simulink model "sim_taes_2023_att"  (R2020a)
settings: Solver=ode4  StartTime=0.0  StopTime=30.0  FixedStep=0.01  RelTol=1e-3
values from neighbouring files (symbols this model uses):
  c1_diff_sigma_bar_w = diag([12; 12; 12])    [init_taes_2023_att.m]
  c1_diff_ui = diag([25; 30; 20])    [init_taes_2023_att.m]
  c2_diff_sigma_bar_w = diag([12; 12; 12])    [init_taes_2023_att.m]
  c2_diff_ui = diag([50; 50; 10])    [init_taes_2023_att.m]
  c3_diff_sigma_bar_w = diag([15; 15; 15])    [init_taes_2023_att.m]
  c3_diff_ui = diag([15; 15; 10])    [init_taes_2023_att.m]
  cw = diag([4.0; 4.0; 4.0])    [init_taes_2023_att.m]
  dw_aa_t = 0.2 * ones(3, 5) + ( 1.0 - 0.2 ) * rand(3, 5)    [init_taes_2023_att.m]
  dw_ff_t = [ 0.4 * ones(1, 5) + ( 1.0 - 0.4 ) * rand(1, 5);                      0.4 * ones(1, 5) + ( 1.0 - 0.4 ) * rand(1, 5);                      0.2 * ones(1, 5) + ( 0.6 - 0.2 ) * rand(1, 5) ]    [init_taes_2023_att.m]
  dw_phi_t = ( - pi / 2 ) * ones(3, 5) + ( pi / 2 - ( - pi / 2 ) ) * rand(3, 5)    [init_taes_2023_att.m]
  dwci_init = zeros(3,5)    [init_taes_2023_att.m]
  h1w = diag([20.0; 20.0; 20.0])    [init_taes_2023_att.m]
  h2w = diag([35.0; 35.0; 35.0])    [init_taes_2023_att.m]
  h3w = diag([30.0; 30.0; 30.0])    [init_taes_2023_att.m]
  Ji = zeros(3,3,NF)    [init_taes_2023_att.m]
  kR = diag([40; 40; 40])    [init_taes_2023_att.m]
  kRtilt = diag([90; 90; 90])    [init_taes_2023_att.m]
  Lamd_diff_sigma_bar_w = 0.5    [init_taes_2023_att.m]
  Lamd_diff_ui = 0.5    [init_taes_2023_att.m]
  mu_d_w = 100    [init_taes_2023_att.m]
  pos0 = zeros(3, 1)    [init_taes_2023_att.m]
  PZ0 = P0(3)    [init_taes_2023_att.m]
  PZ1 = 10    [init_taes_2023_att.m]
  Qci_init = repmat([1;0;0;0],1,NF)    [init_taes_2023_att.m]
  R0 = 4    [init_taes_2023_att.m]
  R1 = 8    [init_taes_2023_att.m]
  Rci_init = zeros(3,3,NF)    [init_taes_2023_att.m]
  Ri_init = zeros(3,3,NF)    [init_taes_2023_att.m]
  Rx2 = 10    [init_taes_2023_att.m]
  Ry2 = 6    [init_taes_2023_att.m]
  Rz2 = 4    [init_taes_2023_att.m]
  T0 = 0    [init_taes_2023_att.m]
  T1 = tseq1    (= 10)    [init_taes_2023_att.m]
  T2 = tseq1 + tseq12 + tseq2    (= 30)    [init_taes_2023_att.m]
  ui_init = zeros(3,NF)    [init_taes_2023_att.m]
  vel0 = zeros(3, 1)    [init_taes_2023_att.m]
  wci_init = zeros(3,5)    [init_taes_2023_att.m]
  zeta_diff_sigma_bar_w = 0.08    [init_taes_2023_att.m]
  zeta_diff_ui = 0.08    [init_taes_2023_att.m]
undefined symbols (not defined in the file or in its folder): cal_frac_squ, p_alfaw1, p_alfaw2, q_alfaw1, q_alfaw2, Qei_init, Qeitilt_init, Qi_init, Rei_init, Reitilt_init, V_Phi_Rei_init, V_Phi_Reitilt_init, wei_init, weitilt_init, wi_init
(part 4 of 4)

== matlab function sim_taes_2023_att/cal Ri agent 5 ==
  data: Ri_5 output; Qi_vec input
function Ri_5 = fcn(Qi_vec)
%%%% 使用罗德里格公式由四元数Qi求解Ri
iiuav = 5;
thetai_tmp = Qi_vec(1,iiuav);
qi_tmp = Qi_vec(2:4,iiuav);
Ri_5 = ((thetai_tmp^2) - (qi_tmp')*qi_tmp) * eye(3,3) ...
            + 2 * qi_tmp * (qi_tmp') ...
            - 2 * thetai_tmp * cal_askew_mat(qi_tmp);

end

== matlab function sim_taes_2023_att/cal Qci agent 1 ==
  data: Qi_vec input; Qci_1 output; Qei_vec input
function Qci_1 = fcn(Qi_vec, Qei_vec)
%%%% 更新期望指令四元数
iiuav = 1;

sigma1 = Qi_vec(1,iiuav);
q1 = Qi_vec(2:4,iiuav);
sigma2 = Qei_vec(1,iiuav);
q2 = -Qei_vec(2:4,iiuav);

sigma = sigma1*sigma2 - (q1')*q2;
q = sigma1*q2 + sigma2*q1 + cal_askew_mat(q1)*q2;
Qci_1 = [sigma; q];

end

== matlab function sim_taes_2023_att/cal Rci agent 1 ==
  data: Rci_1 output; Qci input
function Rci_1 = fcn(Qci)
%%%% 使用罗德里格公式由四元数Qci求解Rci
thetaci_tmp = Qci(1,1);
qci_tmp = Qci(2:4,1);
Rci_1 = ((thetaci_tmp^2) - (qci_tmp')*qci_tmp) * eye(3,3) ...
                + 2 * qci_tmp * (qci_tmp') ...
                - 2 * thetaci_tmp * cal_askew_mat(qci_tmp);

end

== matlab function sim_taes_2023_att/cal Qci agent 2 ==
  data: Qi_vec input; Qci_2 output; Qei_vec input
function Qci_2 = fcn(Qi_vec, Qei_vec)
%%%% 更新期望指令四元数
iiuav = 2;
sigma1 = Qi_vec(1,iiuav);
q1 = Qi_vec(2:4,iiuav);
sigma2 = Qei_vec(1,iiuav);
q2 = -Qei_vec(2:4,iiuav);

sigma = sigma1*sigma2 - (q1')*q2;
q = sigma1*q2 + sigma2*q1 + cal_askew_mat(q1)*q2;
Qci_2 = [sigma; q];

end

== matlab function sim_taes_2023_att/cal Rci agent 2 ==
  data: Rci_2 output; Qci input
function Rci_2 = fcn(Qci)
%%%% 使用罗德里格公式由四元数Qci求解Rci

thetaci_tmp = Qci(1,1);
qci_tmp = Qci(2:4,1);
Rci_2 = ((thetaci_tmp^2) - (qci_tmp')*qci_tmp) * eye(3,3) ...
                + 2 * qci_tmp * (qci_tmp') ...
                - 2 * thetaci_tmp * cal_askew_mat(qci_tmp);

end

== matlab function sim_taes_2023_att/cal Qci agent 3 ==
  data: Qi_vec input; Qci_3 output; Qei_vec input
function Qci_3 = fcn(Qi_vec, Qei_vec)
%%%% 更新期望指令四元数
iiuav = 3;
sigma1 = Qi_vec(1,iiuav);
q1 = Qi_vec(2:4,iiuav);
sigma2 = Qei_vec(1,iiuav);
q2 = -Qei_vec(2:4,iiuav);

sigma = sigma1*sigma2 - (q1')*q2;
q = sigma1*q2 + sigma2*q1 + cal_askew_mat(q1)*q2;
Qci_3 = [sigma; q];

end

== matlab function sim_taes_2023_att/cal differentiator d_sigma_bar_w_hat agent 1/cal sig3 ==
  data: x input; z output; y input
function z = fcn(x, y)
z = x(:) .* sign(y(:));

== matlab function sim_taes_2023_att/cal Rci agent 3 ==
  data: Rci_3 output; Qci input
function Rci_3 = fcn(Qci)
%%%% 使用罗德里格公式由四元数Qci求解Rci
thetaci_tmp = Qci(1,1);
qci_tmp = Qci(2:4,1);
Rci_3 = ((thetaci_tmp^2) - (qci_tmp')*qci_tmp) * eye(3,3) ...
                + 2 * qci_tmp * (qci_tmp') ...
                - 2 * thetaci_tmp * cal_askew_mat(qci_tmp);

end

== matlab function sim_taes_2023_att/cal Qci agent 4 ==
  data: Qi_vec input; Qci_4 output; Qei_vec input
function Qci_4 = fcn(Qi_vec, Qei_vec)
%%%% 更新期望指令四元数
iiuav = 4;
sigma1 = Qi_vec(1,iiuav);
q1 = Qi_vec(2:4,iiuav);
sigma2 = Qei_vec(1,iiuav);
q2 = -Qei_vec(2:4,iiuav);

sigma = sigma1*sigma2 - (q1')*q2;
q = sigma1*q2 + sigma2*q1 + cal_askew_mat(q1)*q2;
Qci_4 = [sigma; q];

end

== matlab function sim_taes_2023_att/cal Rci agent 4 ==
  data: Rci_4 output; Qci input
function Rci_4 = fcn(Qci)
%%%% 使用罗德里格公式由四元数Qci求解Rci
thetaci_tmp = Qci(1,1);
qci_tmp = Qci(2:4,1);
Rci_4 = ((thetaci_tmp^2) - (qci_tmp')*qci_tmp) * eye(3,3) ...
                + 2 * qci_tmp * (qci_tmp') ...
                - 2 * thetaci_tmp * cal_askew_mat(qci_tmp);

end

== matlab function sim_taes_2023_att/cal Qci agent 5 ==
  data: Qi_vec input; Qci_5 output; Qei_vec input
function Qci_5 = fcn(Qi_vec, Qei_vec)
%%%% 更新期望指令四元数
iiuav = 5;
sigma1 = Qi_vec(1,iiuav);
q1 = Qi_vec(2:4,iiuav);
sigma2 = Qei_vec(1,iiuav);
q2 = -Qei_vec(2:4,iiuav);

sigma = sigma1*sigma2 - (q1')*q2;
q = sigma1*q2 + sigma2*q1 + cal_askew_mat(q1)*q2;
Qci_5 = [sigma; q];

end

== matlab function sim_taes_2023_att/cal Rci agent 5 ==
  data: Rci_5 output; Qci_vec input
function Rci_5 = fcn(Qci_vec)
%%%% 使用罗德里格公式由四元数Qci求解Rci
thetaci_tmp = Qci_vec(1,1);
qci_tmp = Qci_vec(2:4,1);
Rci_5 = ((thetaci_tmp^2) - (qci_tmp')*qci_tmp) * eye(3,3) ...
                + 2 * qci_tmp * (qci_tmp') ...
                - 2 * thetaci_tmp * cal_askew_mat(qci_tmp);

end

== matlab function sim_taes_2023_att/combine Qci Rci ==
  data: Qci_1 input; Qci_vec output; Qci_2 input; Qci_3 input; Qci_4 input; Qci_5 input; Rci_1 input; Rci_2 input; Rci_3 input; Rci_4 input; Rci_5 input; Rci_vec output
function [Qci_vec, Rci_vec] = fcn(Qci_1, Qci_2, Qci_3, Qci_4, Qci_5, ...
                                                            Rci_1, Rci_2, Rci_3, Rci_4, Rci_5)
%%%% 合并四元数和姿态旋转矩阵
Qci_vec = zeros(4,5);
Qci_vec(:,1) = Qci_1(:);
Qci_vec(:,2) = Qci_2(:);
Qci_vec(:,3) = Qci_3(:);
Qci_vec(:,4) = Qci_4(:);
Qci_vec(:,5) = Qci_5(:);

Rci_vec = zeros(3,3,5);
Rci_vec(:,:,1) = Rci_1;
Rci_vec(:,:,2) = Rci_2;
Rci_vec(:,:,3) = Rci_3;
Rci_vec(:,:,4) = Rci_4;
Rci_vec(:,:,5) = Rci_5;

== matlab function sim_taes_2023_att/Qeitilt dynam agent 1 ==
  data: Qeitilt_vec input; dQeitilt_1 output; weitilt_vec input
function dQeitilt_1 = fcn(Qeitilt_vec, weitilt_vec)
%%%% 更新四元数误差微分方程
iiuav = 1;

weitilt = weitilt_vec(:,iiuav);
thetaeitilt = Qeitilt_vec(1,iiuav);
qeitilt = Qeitilt_vec(2:4,iiuav);

GammaQeitilt = zeros(4,3);
GammaQeitilt(1,:) = -(qeitilt');
GammaQeitilt(2:4,:) = thetaeitilt*eye(3,3) + cal_askew_mat(qeitilt);
dQeitilt_1 = (1/2)*GammaQeitilt*weitilt;

end

== matlab function sim_taes_2023_att/cal Reitilt agent 1 ==
  data: Reitilt_1 output; Qeitilt_vec input
function Reitilt_1 = fcn(Qeitilt_vec)
%%%% 使用罗德里格公式由四元数Qeitilt求解Reitilt
iiuav = 1;
thetaeitilt_tmp = Qeitilt_vec(1,iiuav);
qeitilt_tmp = Qeitilt_vec(2:4,iiuav);
Reitilt_1 = ((thetaeitilt_tmp^2) - (qeitilt_tmp')*qeitilt_tmp) * eye(3,3) ...
                    + 2 * qeitilt_tmp * (qeitilt_tmp') ...
                    - 2 * thetaeitilt_tmp * cal_askew_mat(qeitilt_tmp);

end

== matlab function sim_taes_2023_att/cal weitilt agent 1 ==
  data: wei_vec input; weitilt_1 output; Reitilt_vec input; wbarei_vec input
function weitilt_1 = fcn(wei_vec, Reitilt_vec, wbarei_vec)
%%%% 更新姿态角速率误差
iiuav = 1;
weitilt_1 = wei_vec(:,iiuav) - (Reitilt_vec(:,:,iiuav)') * wbarei_vec(:,iiuav);

end

== matlab function sim_taes_2023_att/cal differentiator d_sigma_bar_w_hat agent 1/cal sig4 ==
  data: x input; z output; y input
function z = fcn(x, y)
z = x(:) .* sign(y(:));

== matlab function sim_taes_2023_att/Qeitilt dynam agent 2 ==
  data: Qeitilt_vec input; dQeitilt_2 output; weitilt_vec input
function dQeitilt_2 = fcn(Qeitilt_vec, weitilt_vec)
%%%% 更新四元数误差微分方程
iiuav = 2;

weitilt = weitilt_vec(:,iiuav);
thetaeitilt = Qeitilt_vec(1,iiuav);
qeitilt = Qeitilt_vec(2:4,iiuav);

GammaQeitilt = zeros(4,3);
GammaQeitilt(1,:) = -(qeitilt');
GammaQeitilt(2:4,:) = thetaeitilt*eye(3,3) + cal_askew_mat(qeitilt);
dQeitilt_2 = (1/2)*GammaQeitilt*weitilt;

end

== matlab function sim_taes_2023_att/cal Reitilt agent 2 ==
  data: Reitilt_2 output; Qeitilt_vec input
function Reitilt_2 = fcn(Qeitilt_vec)
%%%% 使用罗德里格公式由四元数Qeitilt求解Reitilt
iiuav = 2;
thetaeitilt_tmp = Qeitilt_vec(1,iiuav);
qeitilt_tmp = Qeitilt_vec(2:4,iiuav);
Reitilt_2 = ((thetaeitilt_tmp^2) - (qeitilt_tmp')*qeitilt_tmp) * eye(3,3) ...
                    + 2 * qeitilt_tmp * (qeitilt_tmp') ...
                    - 2 * thetaeitilt_tmp * cal_askew_mat(qeitilt_tmp);

end

== matlab function sim_taes_2023_att/cal weitilt agent 2 ==
  data: wei_vec input; weitilt_2 output; Reitilt_vec input; wbarei_vec input
function weitilt_2 = fcn(wei_vec, Reitilt_vec, wbarei_vec)
%%%% 更新姿态角速率误差
iiuav = 2;
weitilt_2 = wei_vec(:,iiuav) - (Reitilt_vec(:,:,iiuav)') * wbarei_vec(:,iiuav);

end

== matlab function sim_taes_2023_att/Qeitilt dynam agent 3 ==
  data: Qeitilt_vec input; dQeitilt_3 output; weitilt_vec input
function dQeitilt_3 = fcn(Qeitilt_vec, weitilt_vec)
%%%% 更新四元数误差微分方程
iiuav = 3;

weitilt = weitilt_vec(:,iiuav);
thetaeitilt = Qeitilt_vec(1,iiuav);
qeitilt = Qeitilt_vec(2:4,iiuav);

GammaQeitilt = zeros(4,3);
GammaQeitilt(1,:) = -(qeitilt');
GammaQeitilt(2:4,:) = thetaeitilt*eye(3,3) + cal_askew_mat(qeitilt);
dQeitilt_3 = (1/2)*GammaQeitilt*weitilt;

end

== matlab function sim_taes_2023_att/cal Reitilt agent 3 ==
  data: Reitilt_3 output; Qeitilt_vec input
function Reitilt_3 = fcn(Qeitilt_vec)
%%%% 使用罗德里格公式由四元数Qeitilt求解Reitilt
iiuav = 3;
thetaeitilt_tmp = Qeitilt_vec(1,iiuav);
qeitilt_tmp = Qeitilt_vec(2:4,iiuav);
Reitilt_3 = ((thetaeitilt_tmp^2) - (qeitilt_tmp')*qeitilt_tmp) * eye(3,3) ...
                    + 2 * qeitilt_tmp * (qeitilt_tmp') ...
                    - 2 * thetaeitilt_tmp * cal_askew_mat(qeitilt_tmp);

end

== matlab function sim_taes_2023_att/cal weitilt agent 3 ==
  data: wei_vec input; weitilt_3 output; Reitilt_vec input; wbarei_vec input
function weitilt_3 = fcn(wei_vec, Reitilt_vec, wbarei_vec)
%%%% 更新姿态角速率误差
iiuav = 3;
weitilt_3 = wei_vec(:,iiuav) - (Reitilt_vec(:,:,iiuav)') * wbarei_vec(:,iiuav);

end

== matlab function sim_taes_2023_att/Qeitilt dynam agent 4 ==
  data: Qeitilt_vec input; dQeitilt_4 output; weitilt_vec input
function dQeitilt_4 = fcn(Qeitilt_vec, weitilt_vec)
%%%% 更新四元数误差微分方程
iiuav = 4;

weitilt = weitilt_vec(:,iiuav);
thetaeitilt = Qeitilt_vec(1,iiuav);
qeitilt = Qeitilt_vec(2:4,iiuav);

GammaQeitilt = zeros(4,3);
GammaQeitilt(1,:) = -(qeitilt');
GammaQeitilt(2:4,:) = thetaeitilt*eye(3,3) + cal_askew_mat(qeitilt);
dQeitilt_4 = (1/2)*GammaQeitilt*weitilt;

end

== matlab function sim_taes_2023_att/cal Reitilt agent 4 ==
  data: Reitilt_4 output; Qeitilt_vec input
function Reitilt_4 = fcn(Qeitilt_vec)
%%%% 使用罗德里格公式由四元数Qeitilt求解Reitilt
iiuav = 4;
thetaeitilt_tmp = Qeitilt_vec(1,iiuav);
qeitilt_tmp = Qeitilt_vec(2:4,iiuav);
Reitilt_4 = ((thetaeitilt_tmp^2) - (qeitilt_tmp')*qeitilt_tmp) * eye(3,3) ...
                    + 2 * qeitilt_tmp * (qeitilt_tmp') ...
                    - 2 * thetaeitilt_tmp * cal_askew_mat(qeitilt_tmp);

end

== matlab function sim_taes_2023_att/cal weitilt agent 4 ==
  data: wei_vec input; weitilt_4 output; Reitilt_vec input; wbarei_vec input
function weitilt_4 = fcn(wei_vec, Reitilt_vec, wbarei_vec)
%%%% 更新姿态角速率误差
iiuav = 4;
weitilt_4 = wei_vec(:,iiuav) - (Reitilt_vec(:,:,iiuav)') * wbarei_vec(:,iiuav);

end

== matlab function sim_taes_2023_att/Qeitilt dynam agent 5 ==
  data: Qeitilt_vec input; dQeitilt_5 output; weitilt_vec input
function dQeitilt_5 = fcn(Qeitilt_vec, weitilt_vec)
%%%% 更新四元数误差微分方程
iiuav = 5;

weitilt = weitilt_vec(:,iiuav);
thetaeitilt = Qeitilt_vec(1,iiuav);
qeitilt = Qeitilt_vec(2:4,iiuav);

GammaQeitilt = zeros(4,3);
GammaQeitilt(1,:) = -(qeitilt');
GammaQeitilt(2:4,:) = thetaeitilt*eye(3,3) + cal_askew_mat(qeitilt);
dQeitilt_5 = (1/2)*GammaQeitilt*weitilt;

end

== matlab function sim_taes_2023_att/cal differentiator d_sigma_bar_w_hat agent 1/cal sig5 ==
  data: x input; z output; y input
function z = fcn(x, y)
z = x(:) .* sign(y(:));

== matlab function sim_taes_2023_att/cal Reitilt agent 5 ==
  data: Reitilt_5 output; Qeitilt_vec input
function Reitilt_5 = fcn(Qeitilt_vec)
%%%% 使用罗德里格公式由四元数Qeitilt求解Reitilt
iiuav = 5;
thetaeitilt_tmp = Qeitilt_vec(1,iiuav);
qeitilt_tmp = Qeitilt_vec(2:4,iiuav);
Reitilt_5 = ((thetaeitilt_tmp^2) - (qeitilt_tmp')*qeitilt_tmp) * eye(3,3) ...
                    + 2 * qeitilt_tmp * (qeitilt_tmp') ...
                    - 2 * thetaeitilt_tmp * cal_askew_mat(qeitilt_tmp);

end

== matlab function sim_taes_2023_att/cal weitilt agent 5 ==
  data: wei_vec input; weitilt_5 output; Reitilt_vec input; wbarei_vec input
function weitilt_5 = fcn(wei_vec, Reitilt_vec, wbarei_vec)
%%%% 更新姿态角速率误差
iiuav = 5;
weitilt_5 = wei_vec(:,iiuav) - (Reitilt_vec(:,:,iiuav)') * wbarei_vec(:,iiuav);

end

== matlab function sim_taes_2023_att/combine weitilt Qeitilt Reitilt ==
  data: weitilt_1 input; weitilt_vec output; weitilt_2 input; weitilt_3 input; weitilt_4 input; weitilt_5 input; Qeitilt_1 input; Qeitilt_2 input; Qeitilt_3 input; Qeitilt_4 input; Qeitilt_5 input; Reitilt_1 input; Reitilt_2 input; Reitilt_3 input; Reitilt_4 input; Reitilt_5 input; Qeitilt_vec output; Reitilt_vec output
function [weitilt_vec, Qeitilt_vec, Reitilt_vec] = fcn(weitilt_1, weitilt_2, weitilt_3, weitilt_4, weitilt_5, ...
                                                                                            Qeitilt_1, Qeitilt_2, Qeitilt_3, Qeitilt_4, Qeitilt_5, ...
                                                                                            Reitilt_1, Reitilt_2, Reitilt_3, Reitilt_4, Reitilt_5)
%%%% 合并辅助姿态角速率误差/辅助四元数误差/辅助姿态旋转矩阵误差
weitilt_vec = zeros(3,5);
weitilt_vec(:,1) = weitilt_1(:);
weitilt_vec(:,2) = weitilt_2(:);
weitilt_vec(:,3) = weitilt_3(:);
weitilt_vec(:,4) = weitilt_4(:);
weitilt_vec(:,5) = weitilt_5(:);

Qeitilt_vec = zeros(4,5);
Qeitilt_vec(:,1) = Qeitilt_1(:);
Qeitilt_vec(:,2) = Qeitilt_2(:);
Qeitilt_vec(:,3) = Qeitilt_3(:);
Qeitilt_vec(:,4) = Qeitilt_4(:);
Qeitilt_vec(:,5) = Qeitilt_5(:);

Reitilt_vec = zeros(3,3,5);
Reitilt_vec(:,:,1) = Reitilt_1;
Reitilt_vec(:,:,2) = Reitilt_2;
Reitilt_vec(:,:,3) = Reitilt_3;
Reitilt_vec(:,:,4) = Reitilt_4;
Reitilt_vec(:,:,5) = Reitilt_5;

== matlab function sim_taes_2023_att/cal error dw_tilt ==
  data: dw_vec input; dw_hat_vec input; dw_tilt_vec output
function dw_tilt_vec = fcn(dw_vec, dw_hat_vec)
%%%% 计算扰动观测误差dw_tilt
dw_tilt_vec = zeros(3,5);
for iiuav = 1:5
    dw_tilt_vec(:,iiuav) = dw_vec(:,iiuav) - dw_hat_vec(:,iiuav);
end

== matlab function sim_taes_2023_att/combine Qci Rci1 ==
  data: V_Phi_Rei_1 input; V_Phi_Rei_vec output; V_Phi_Rei_2 input; V_Phi_Rei_3 input; V_Phi_Rei_4 input; V_Phi_Rei_5 input; V_Phi_Reitilt_1 input; V_Phi_Reitilt_2 input; V_Phi_Reitilt_3 input; V_Phi_Reitilt_4 input; V_Phi_Reitilt_5 input; V_Phi_Reitilt_vec output
function [V_Phi_Rei_vec, V_Phi_Reitilt_vec] = fcn(V_Phi_Rei_1, V_Phi_Rei_2, V_Phi_Rei_3, V_Phi_Rei_4, V_Phi_Rei_5, ...
                                                                                        V_Phi_Reitilt_1, V_Phi_Reitilt_2, V_Phi_Reitilt_3, V_Phi_Reitilt_4, V_Phi_Reitilt_5)
%%%% 合并LogSO3空间的辅助姿态误差向量
V_Phi_Rei_vec = [V_Phi_Rei_1(:), V_Phi_Rei_2(:), V_Phi_Rei_3(:), V_Phi_Rei_4(:), V_Phi_Rei_5(:)];
V_Phi_Reitilt_vec = [V_Phi_Reitilt_1(:), V_Phi_Reitilt_2(:), V_Phi_Reitilt_3(:), V_Phi_Reitilt_4(:), V_Phi_Reitilt_5(:)];

== matlab function sim_taes_2023_att/depart Qe1 ==
  data: y output; x input
function y = fcn(x)
y = x(:,1);

end

== matlab function sim_taes_2023_att/depart Qe2 ==
  data: y output; x input
function y = fcn(x)
y = x(:,2);

end

== matlab function sim_taes_2023_att/cal differentiator d_sigma_bar_w_hat agent 1/trans to column20 ==
  data: x input; y output
function y = fcn(x)
y = x(:);

== matlab function sim_taes_2023_att/depart Qe3 ==
  data: y output; x input
function y = fcn(x)
y = x(:,3);

end

== matlab function sim_taes_2023_att/depart Qe4 ==
  data: y output; x input
function y = fcn(x)
y = x(:,4);

end

== matlab function sim_taes_2023_att/depart Qe5 ==
  data: y output; x input
function y = fcn(x)
y = x(:,5);

end

== matlab function sim_taes_2023_att/depart Qe5tilt ==
  data: y output; x input
function y = fcn(x)
y = x(:,5);

end

== matlab function sim_taes_2023_att/depart Qe1tilt ==
  data: y output; x input
function y = fcn(x)
y = x(:,1);

end

== matlab function sim_taes_2023_att/depart Qe2tilt ==
  data: y output; x input
function y = fcn(x)
y = x(:,2);

end

== matlab function sim_taes_2023_att/depart Qe3tilt ==
  data: y output; x input
function y = fcn(x)
y = x(:,3);

end

== matlab function sim_taes_2023_att/depart Qe4tilt ==
  data: y output; x input
function y = fcn(x)
y = x(:,4);

end

== matlab function sim_taes_2023_att/depart we1 ==
  data: y output; x input
function y = fcn(x)
y = x(:,1);

end

== matlab function sim_taes_2023_att/depart we2 ==
  data: y output; x input
function y = fcn(x)
y = x(:,2);

end

== matlab function sim_taes_2023_att/cal differentiator d_sigma_bar_w_hat agent 1/trans to column23 ==
  data: x input; y output
function y = fcn(x)
y = x(:);

== matlab function sim_taes_2023_att/depart we3 ==
  data: y output; x input
function y = fcn(x)
y = x(:,3);

end

== matlab function sim_taes_2023_att/depart we4 ==
  data: y output; x input
function y = fcn(x)
y = x(:,4);

end

== matlab function sim_taes_2023_att/depart we5 ==
  data: y output; x input
function y = fcn(x)
y = x(:,5);

end

== matlab function sim_taes_2023_att/depart we5tilt ==
  data: y output; x input
function y = fcn(x)
y = x(:,5);

end

== matlab function sim_taes_2023_att/depart we1tilt ==
  data: y output; x input
function y = fcn(x)
y = x(:,1);

end

== matlab function sim_taes_2023_att/depart we2tilt ==
  data: y output; x input
function y = fcn(x)
y = x(:,2);

end

== matlab function sim_taes_2023_att/depart we3tilt ==
  data: y output; x input
function y = fcn(x)
y = x(:,3);

end

== matlab function sim_taes_2023_att/depart we4tilt ==
  data: y output; x input
function y = fcn(x)
y = x(:,4);

end

== matlab function sim_taes_2023_att/depart V_Phi_Re5 ==
  data: y output; x input
function y = fcn(x)
y = x(:,5);

end

== matlab function sim_taes_2023_att/depart V_Phi_Re1 ==
  data: y output; x input
function y = fcn(x)
y = x(:,1);

end

== matlab function sim_taes_2023_att/cal differentiator d_sigma_bar_w_hat agent 2/cal differentiator ==
  data: c1 input; d_sigma_bar_v_hat output; d_dsigma_bar_v_hat output; d_d2sigma_bar_v_hat output; c2 input; c3 input; chi_t input; sigma_bar_v_sig_1 input; sigma_bar_v_sig_2 input; sigma_bar_v_sig_3 input; sigma_bar_v_sig_4 input; sigma_bar_v_sig_5 input; sigma_bar_v_sig_6 input; d_sigma_bar_v_hat input; d2_sigma_bar_v_hat input
function [d_sigma_bar_v_hat, d_dsigma_bar_v_hat, d_d2sigma_bar_v_hat] = fcn(c1, c2, c3, chi_t, sigma_bar_v_sig_1, sigma_bar_v_sig_2, sigma_bar_v_sig_3, ...
                                                                                                                                                sigma_bar_v_sig_4, sigma_bar_v_sig_5, sigma_bar_v_sig_6, d_sigma_bar_v_hat, d2_sigma_bar_v_hat)
d_d2sigma_bar_v_hat = -chi_t .* c1 * sigma_bar_v_sig_1(:) - (1 - chi_t) .* c1 * sigma_bar_v_sig_2(:);
d_dsigma_bar_v_hat = -chi_t .* c2 * sigma_bar_v_sig_3(:) - (1 - chi_t) .* c2 * sigma_bar_v_sig_4(:) + d2_sigma_bar_v_hat(:);
d_sigma_bar_v_hat = -chi_t .* c3 * sigma_bar_v_sig_5(:) - (1 - chi_t) .* c3 * sigma_bar_v_sig_6(:) + d_sigma_bar_v_hat(:);

== matlab function sim_taes_2023_att/depart V_Phi_Re2 ==
  data: y output; x input
function y = fcn(x)
y = x(:,2);

end

== matlab function sim_taes_2023_att/depart V_Phi_Re3 ==
  data: y output; x input
function y = fcn(x)
y = x(:,3);

end

== matlab function sim_taes_2023_att/depart V_Phi_Re4 ==
  data: y output; x input
function y = fcn(x)
y = x(:,4);

end

== matlab function sim_taes_2023_att/depart V_Phi_Re5tilt ==
  data: y output; x input
function y = fcn(x)
y = x(:,5);

end

== matlab function sim_taes_2023_att/depart V_Phi_Re1tilt ==
  data: y output; x input
function y = fcn(x)
y = x(:,1);

end

== matlab function sim_taes_2023_att/depart V_Phi_Re2tilt ==
  data: y output; x input
function y = fcn(x)
y = x(:,2);

end

== matlab function sim_taes_2023_att/depart V_Phi_Re3tilt ==
  data: y output; x input
function y = fcn(x)
y = x(:,3);

end

== matlab function sim_taes_2023_att/depart V_Phi_Re4tilt ==
  data: y output; x input
function y = fcn(x)
y = x(:,4);

end

== matlab function sim_taes_2023_att/depart dw1 dw_hat_1 ==
  data: y1 output; x1 input; x2 input; y2 output
function [y1, y2] = fcn(x1, x2)
iiuav = 1;
y1 = x1(:,iiuav);
y2 = x2(:,iiuav);

end

== matlab function sim_taes_2023_att/depart dw2 dw_hat_2 ==
  data: y1 output; x1 input; x2 input; y2 output
function [y1, y2] = fcn(x1, x2)
iiuav = 2;
y1 = x1(:,iiuav);
y2 = x2(:,iiuav);

end

== matlab function sim_taes_2023_att/depart dw3 dw_hat_3 ==
  data: y1 output; x1 input; x2 input; y2 output
function [y1, y2] = fcn(x1, x2)
iiuav = 3;
y1 = x1(:,iiuav);
y2 = x2(:,iiuav);

end

== matlab function sim_taes_2023_att/depart dw4 dw_hat_4 ==
  data: y1 output; x1 input; x2 input; y2 output
function [y1, y2] = fcn(x1, x2)
iiuav = 4;
y1 = x1(:,iiuav);
y2 = x2(:,iiuav);

end

== matlab function sim_taes_2023_att/depart dw4 dw_hat_1 ==
  data: y1 output; x1 input; x2 input; y2 output
function [y1, y2] = fcn(x1, x2)
iiuav = 4;
y1 = x1(:,iiuav);
y2 = x2(:,iiuav);

end

== matlab function sim_taes_2023_att/depart Qc1 ==
  data: y output; x input
function y = fcn(x)
y = x(:,1);

end

== matlab function sim_taes_2023_att/depart Qc2 ==
  data: y output; x input
function y = fcn(x)
y = x(:,2);

end

== matlab function sim_taes_2023_att/depart Qc3 ==
  data: y output; x input
function y = fcn(x)
y = x(:,3);

end

== matlab function sim_taes_2023_att/depart Qc4 ==
  data: y output; x input
function y = fcn(x)
y = x(:,4);

end

== matlab function sim_taes_2023_att/depart Qc5 ==
  data: y output; x input
function y = fcn(x)
y = x(:,5);

end

== matlab function sim_taes_2023_att/depart wc1 ==
  data: y output; x input
function y = fcn(x)
y = x(:,1);

end

== matlab function sim_taes_2023_att/depart wc2 ==
  data: y output; x input
function y = fcn(x)
y = x(:,2);

end

== matlab function sim_taes_2023_att/depart wc3 ==
  data: y output; x input
function y = fcn(x)
y = x(:,3);

end

== matlab function sim_taes_2023_att/depart wc4 ==
  data: y output; x input
function y = fcn(x)
y = x(:,4);

end

== matlab function sim_taes_2023_att/depart wc5 ==
  data: y output; x input
function y = fcn(x)
y = x(:,5);

end

== matlab function sim_taes_2023_att/combine tau1 ==
  data: dw_1 input; dw_vec output; dw_2 input; dw_3 input; dw_4 input; dw_5 input
function dw_vec = fcn(dw_1, dw_2, dw_3, dw_4, dw_5)
%%%% 合并辅助姿态角速率
dw_vec = [dw_1(:), dw_2(:), dw_3(:), dw_4(:), dw_5(:)];

== matlab function sim_taes_2023_att/generate angular rate disturbance agent 1 ==
  data: dw_1 output; dw_aa_t input; dw_ff_t input; dw_phi_t input; t input
function dw_1 = fcn(dw_aa_t, dw_ff_t, dw_phi_t, t)
%%%% 姿态动力学方程中的扰动项设置
epsil_t = zeros(3, 1);

for kk = 1:5
    epsil_t = epsil_t + dw_aa_t(:, kk) .* sin( 2 * pi * dw_ff_t(:, kk) * t + dw_phi_t(:, kk) );
end

dw_1 = [ epsil_t(1) + 1.6 * sin( 0.4 * t ) + 2.0 * cos( 0.5 * t ) + 1.4 * sin( 0.7 * t ) ...
                + 4 * exp( -0.1 * t ) * sin( 0.8 * t ) + 3 / ( 1 + exp( -0.2 * ( t - 15 ) ) ); ...
                epsil_t(2) + 1.2 * sin( 0.2 * t ) + 3 * cos( 0.4 * t ) + 0.8 * sin( 0.6 * t ) ...
                + 2 * exp( -0.15 * t ) * cos( 1.2 * t ) + 3 / ( 1 + exp( -0.3 * ( t - 25 ) ) ); ...
                epsil_t(3) + 1.8 * sin( 0.2 * t ) + 1.6 * sin( 0.3 * t ) + 1.6 * cos( 0.4 * t ) ...
                + 4 * exp( -0.05 * t ) * sin( 0.5 * t + pi / 4 ) + 3 / ( 1 + exp( -0.5 * ( t - 20 ) ) ) ];

== matlab function sim_taes_2023_att/generate angular rate disturbance agent 2 ==
  data: dw_2 output; dw_aa_t input; dw_ff_t input; dw_phi_t input; t input
function dw_2 = fcn(dw_aa_t, dw_ff_t, dw_phi_t, t)
%%%% 姿态动力学方程中的扰动项设置
epsil_t = zeros(3, 1);

for kk = 1:5
    epsil_t = epsil_t + dw_aa_t(:, kk) .* sin( 2 * pi * dw_ff_t(:, kk) * t + dw_phi_t(:, kk) );
end

dw_2 = [ epsil_t(1) + 1.6 * sin( 0.2 * t ) + 2.0 * cos( 0.3 * t ) + 1.4 * sin( 0.5 * t ) ...
                + 4 * exp( -0.1 * t ) * sin( 0.5 * t ) + 3 / ( 1 + exp( -0.2 * ( t - 15 ) ) ); ...
                epsil_t(2) + 1.2 * sin( 0.1 * t ) + 3 * cos( 0.2 * t ) + 0.8 * sin( 0.4 * t ) ...
                + 2 * exp( -0.15 * t ) * cos( 0.6 * t ) + 3 / ( 1 + exp( -0.3 * ( t - 25 ) ) ); ...
                epsil_t(3) + 1.8 * sin( 0.1 * t ) + 1.6 * sin( 0.2 * t ) + 1.6 * cos( 0.3 * t ) ...
                + 4 * exp( -0.05 * t ) * sin( 0.4 * t + pi / 4 ) + 3 / ( 1 + exp( -0.5 * ( t - 20 ) ) ) ];

== matlab function sim_taes_2023_att/cal differentiator d_sigma_bar_w_hat agent 2/cal sig ==
  data: x input; z output; y input
function z = fcn(x, y)
z = x(:) .* sign(y(:));

== matlab function sim_taes_2023_att/generate angular rate disturbance agent 3 ==
  data: dw_3 output; dw_aa_t input; dw_ff_t input; dw_phi_t input; t input
function dw_3 = fcn(dw_aa_t, dw_ff_t, dw_phi_t, t)
%%%% 姿态动力学方程中的扰动项设置
epsil_t = zeros(3, 1);

for kk = 1:5
    epsil_t = epsil_t + dw_aa_t(:, kk) .* sin( 2 * pi * dw_ff_t(:, kk) * t + dw_phi_t(:, kk) );
end

dw_3 = [ epsil_t(1) + 1.6 * sin( 0.2 * t ) + 2.0 * cos( 0.3 * t ) + 1.4 * sin( 0.5 * t ) ...
                + 4 * exp( -0.1 * t ) * sin( 0.5 * t ) + 3 / ( 1 + exp( -0.2 * ( t - 15 ) ) ); ...
                epsil_t(2) + 1.2 * sin( 0.1 * t ) + 3 * cos( 0.2 * t ) + 0.8 * sin( 0.4 * t ) ...
                + 2 * exp( -0.15 * t ) * cos( 0.6 * t ) + 3 / ( 1 + exp( -0.3 * ( t - 25 ) ) ); ...
                epsil_t(3) + 1.8 * sin( 0.1 * t ) + 1.6 * sin( 0.2 * t ) + 1.6 * cos( 0.3 * t ) ...
                + 4 * exp( -0.05 * t ) * sin( 0.4 * t + pi / 4 ) + 3 / ( 1 + exp( -0.5 * ( t - 20 ) ) ) ];

== matlab function sim_taes_2023_att/generate angular rate disturbance agent 4 ==
  data: dw_4 output; dw_aa_t input; dw_ff_t input; dw_phi_t input; t input
function dw_4 = fcn(dw_aa_t, dw_ff_t, dw_phi_t, t)
%%%% 姿态动力学方程中的扰动项设置
epsil_t = zeros(3, 1);

for kk = 1:5
    epsil_t = epsil_t + dw_aa_t(:, kk) .* sin( 2 * pi * dw_ff_t(:, kk) * t + dw_phi_t(:, kk) );
end

dw_4 = [ epsil_t(1) + 1.6 * sin( 0.2 * t ) + 2.0 * cos( 0.3 * t ) + 1.4 * sin( 0.5 * t ) ...
                + 4 * exp( -0.1 * t ) * sin( 0.5 * t ) + 3 / ( 1 + exp( -0.2 * ( t - 15 ) ) ); ...
                epsil_t(2) + 1.2 * sin( 0.1 * t ) + 3 * cos( 0.2 * t ) + 0.8 * sin( 0.4 * t ) ...
                + 2 * exp( -0.15 * t ) * cos( 0.6 * t ) + 3 / ( 1 + exp( -0.3 * ( t - 25 ) ) ); ...
                epsil_t(3) + 1.8 * sin( 0.1 * t ) + 1.6 * sin( 0.2 * t ) + 1.6 * cos( 0.3 * t ) ...
                + 4 * exp( -0.05 * t ) * sin( 0.4 * t + pi / 4 ) + 3 / ( 1 + exp( -0.5 * ( t - 20 ) ) ) ];

== matlab function sim_taes_2023_att/generate angular rate disturbance agent 5 ==
  data: dw_5 output; dw_aa_t input; dw_ff_t input; dw_phi_t input; t input
function dw_5 = fcn(dw_aa_t, dw_ff_t, dw_phi_t, t)
%%%% 姿态动力学方程中的扰动项设置
epsil_t = zeros(3, 1);

for kk = 1:5
    epsil_t = epsil_t + dw_aa_t(:, kk) .* sin( 2 * pi * dw_ff_t(:, kk) * t + dw_phi_t(:, kk) );
end

dw_5 = [ epsil_t(1) + 1.6 * sin( 0.2 * t ) + 2.0 * cos( 0.3 * t ) + 1.4 * sin( 0.5 * t ) ...
                + 4 * exp( -0.1 * t ) * sin( 0.5 * t ) + 3 / ( 1 + exp( -0.2 * ( t - 15 ) ) ); ...
                epsil_t(2) + 1.2 * sin( 0.1 * t ) + 3 * cos( 0.2 * t ) + 0.8 * sin( 0.4 * t ) ...
                + 2 * exp( -0.15 * t ) * cos( 0.6 * t ) + 3 / ( 1 + exp( -0.3 * ( t - 25 ) ) ); ...
                epsil_t(3) + 1.8 * sin( 0.1 * t ) + 1.6 * sin( 0.2 * t ) + 1.6 * cos( 0.3 * t ) ...
                + 4 * exp( -0.05 * t ) * sin( 0.4 * t + pi / 4 ) + 3 / ( 1 + exp( -0.5 * ( t - 20 ) ) ) ];

== matlab function sim_taes_2023_att/combine norminal formation control input ==
  data: ui_1 input; ui_vec output; ui_2 input; ui_3 input; ui_4 input; ui_5 input
function ui_vec = fcn(ui_1, ui_2, ui_3, ui_4, ui_5)
%%%% 合并领导者编队跟踪误差结果
ui_vec = [ui_1(:), ui_2(:), ui_3(:), ui_4(:), ui_5(:)];

== matlab function sim_taes_2023_att/control input generator agent 1 ==
  data: u0 input; ui output
function ui  = fcn(u0)
%%%% 给出领导者参考加速度控制输入
g0 = 9.80663;
e3 = [0;0;1];

ui = g0 * e3 + u0(:);

== matlab function sim_taes_2023_att/control input generator agent 2 ==
  data: u0 input; ui output
function ui  = fcn(u0)
%%%% 给出领导者参考加速度控制输入
g0 = 9.80663;
e3 = [0;0;1];

ui = g0 * e3 + u0(:);

== matlab function sim_taes_2023_att/control input generator agent 3 ==
  data: u0 input; ui output
function ui  = fcn(u0)
%%%% 给出领导者参考加速度控制输入
g0 = 9.80663;
e3 = [0;0;1];

ui = g0 * e3 + u0(:);

== matlab function sim_taes_2023_att/control input generator agent 4 ==
  data: u0 input; ui output
function ui  = fcn(u0)
%%%% 给出领导者参考加速度控制输入
g0 = 9.80663;
e3 = [0;0;1];

ui = g0 * e3 + u0(:);

== matlab function sim_taes_2023_att/control input generator agent 5 ==
  data: u0 input; ui output
function ui  = fcn(u0)
%%%% 给出领导者参考加速度控制输入
g0 = 9.80663;
e3 = [0;0;1];

ui = g0 * e3 + u0(:);

== matlab function sim_taes_2023_att/cal differentiator d_sigma_bar_w_hat agent 2/cal sig1 ==
  data: x input; z output; y input
function z = fcn(x, y)
z = x(:) .* sign(y(:));

== matlab function sim_taes_2023_att/cal differentiator d_sigma_bar_w_hat agent 2/cal sig2 ==
  data: x input; z output; y input
function z = fcn(x, y)
z = x(:) .* sign(y(:));

== matlab function sim_taes_2023_att/cal differentiator d_sigma_bar_w_hat agent 2/cal sig3 ==
  data: x input; z output; y input
function z = fcn(x, y)
z = x(:) .* sign(y(:));

== matlab function sim_taes_2023_att/cal differentiator d_sigma_bar_w_hat agent 2/cal sig4 ==
  data: x input; z output; y input
function z = fcn(x, y)
z = x(:) .* sign(y(:));

== matlab function sim_taes_2023_att/cal differentiator d_sigma_bar_w_hat agent 2/cal sig5 ==
  data: x input; z output; y input
function z = fcn(x, y)
z = x(:) .* sign(y(:));

== matlab function sim_taes_2023_att/cal differentiator d_sigma_bar_w_hat agent 2/choose sigma_bar_w ==
  data: x input; y output
function y = fcn(x)
iiuav = 2;
y = x(:,iiuav);

== matlab function sim_taes_2023_att/cal differentiator d_sigma_bar_w_hat agent 2/trans to column20 ==
  data: x input; y output
function y = fcn(x)
y = x(:);

== matlab function sim_taes_2023_att/cal differentiator d_sigma_bar_w_hat agent 2/trans to column21 ==
  data: x input; y output
function y = fcn(x)
y = x(:);

== matlab function sim_taes_2023_att/cal differentiator d_sigma_bar_w_hat agent 2/trans to column22 ==
  data: x input; y output
function y = fcn(x)
y = x(:);

== matlab function sim_taes_2023_att/cal differentiator d_sigma_bar_w_hat agent 2/trans to column23 ==
  data: x input; y output
function y = fcn(x)
y = x(:);

== matlab function sim_taes_2023_att/cal differentiator d_sigma_bar_w_hat agent 2/trans to column24 ==
  data: x input; y output
function y = fcn(x)
y = x(:);

== matlab function sim_taes_2023_att/cal differentiator d_sigma_bar_w_hat agent 2/trans to column25 ==
  data: x input; y output
function y = fcn(x)
y = x(:);

== matlab function sim_taes_2023_att/cal differentiator d_sigma_bar_w_hat agent 3/cal differentiator ==
  data: c1 input; d_sigma_bar_v_hat output; d_dsigma_bar_v_hat output; d_d2sigma_bar_v_hat output; c2 input; c3 input; chi_t input; sigma_bar_v_sig_1 input; sigma_bar_v_sig_2 input; sigma_bar_v_sig_3 input; sigma_bar_v_sig_4 input; sigma_bar_v_sig_5 input; sigma_bar_v_sig_6 input; d_sigma_bar_v_hat input; d2_sigma_bar_v_hat input
function [d_sigma_bar_v_hat, d_dsigma_bar_v_hat, d_d2sigma_bar_v_hat] = fcn(c1, c2, c3, chi_t, sigma_bar_v_sig_1, sigma_bar_v_sig_2, sigma_bar_v_sig_3, ...
                                                                                                                                                sigma_bar_v_sig_4, sigma_bar_v_sig_5, sigma_bar_v_sig_6, d_sigma_bar_v_hat, d2_sigma_bar_v_hat)
d_d2sigma_bar_v_hat = -chi_t .* c1 * sigma_bar_v_sig_1(:) - (1 - chi_t) .* c1 * sigma_bar_v_sig_2(:);
d_dsigma_bar_v_hat = -chi_t .* c2 * sigma_bar_v_sig_3(:) - (1 - chi_t) .* c2 * sigma_bar_v_sig_4(:) + d2_sigma_bar_v_hat(:);
d_sigma_bar_v_hat = -chi_t .* c3 * sigma_bar_v_sig_5(:) - (1 - chi_t) .* c3 * sigma_bar_v_sig_6(:) + d_sigma_bar_v_hat(:);

== matlab function sim_taes_2023_att/cal differentiator d_sigma_bar_w_hat agent 3/cal sig ==
  data: x input; z output; y input
function z = fcn(x, y)
z = x(:) .* sign(y(:));

== matlab function sim_taes_2023_att/cal differentiator d_sigma_bar_w_hat agent 3/cal sig1 ==
  data: x input; z output; y input
function z = fcn(x, y)
z = x(:) .* sign(y(:));

== matlab function sim_taes_2023_att/cal d_theta_hat ==
  data: c1 input; d_ui_hat output; d_dui_hat output; d_d2ui_hat output; c2 input; c3 input; chi_t input; ui_sig_1 input; ui_sig_2 input; ui_sig_3 input; ui_sig_4 input; ui_sig_5 input; ui_sig_6 input; dui_hat input; d2ui_hat input
function [d_ui_hat, d_dui_hat, d_d2ui_hat] = fcn(c1, c2, c3, chi_t, ui_sig_1, ui_sig_2, ui_sig_3, ...
                                                                                        ui_sig_4, ui_sig_5, ui_sig_6, dui_hat, d2ui_hat)
d_d2ui_hat = -chi_t .* c1 * ui_sig_1(:) - (1 - chi_t) .* c1 * ui_sig_2(:);
d_dui_hat = -chi_t .* c2 * ui_sig_3(:) - (1 - chi_t) .* c2 * ui_sig_4(:) + d2ui_hat(:);
d_ui_hat = -chi_t .* c3 * ui_sig_5(:) - (1 - chi_t) .* c3 * ui_sig_6(:) + dui_hat(:);

== matlab function sim_taes_2023_att/cal differentiator d_sigma_bar_w_hat agent 3/cal sig2 ==
  data: x input; z output; y input
function z = fcn(x, y)
z = x(:) .* sign(y(:));

== matlab function sim_taes_2023_att/cal differentiator d_sigma_bar_w_hat agent 3/cal sig3 ==
  data: x input; z output; y input
function z = fcn(x, y)
z = x(:) .* sign(y(:));

== matlab function sim_taes_2023_att/cal differentiator d_sigma_bar_w_hat agent 3/cal sig4 ==
  data: x input; z output; y input
function z = fcn(x, y)
z = x(:) .* sign(y(:));

== matlab function sim_taes_2023_att/cal differentiator d_sigma_bar_w_hat agent 3/cal sig5 ==
  data: x input; z output; y input
function z = fcn(x, y)
z = x(:) .* sign(y(:));

== matlab function sim_taes_2023_att/cal differentiator d_sigma_bar_w_hat agent 3/choose sigma_bar_w ==
  data: x input; y output
function y = fcn(x)
iiuav = 3;
y = x(:,iiuav);

== matlab function sim_taes_2023_att/cal differentiator d_sigma_bar_w_hat agent 3/trans to column20 ==
  data: x input; y output
function y = fcn(x)
y = x(:);

== matlab function sim_taes_2023_att/cal sig ==
  data: x input; z output; y input
function z = fcn(x, y)
z = x(:) .* sign(y(:));

== matlab function sim_taes_2023_att/cal sig1 ==
  data: x input; z output; y input
function z = fcn(x, y)
z = x(:) .* sign(y(:));

== matlab function sim_taes_2023_att/cal sig2 ==
  data: x input; z output; y input
function z = fcn(x, y)
z = x(:) .* sign(y(:));

== matlab function sim_taes_2023_att/cal sig3 ==
  data: x input; z output; y input
function z = fcn(x, y)
z = x(:) .* sign(y(:));

== matlab function sim_taes_2023_att/cal sig4 ==
  data: x input; z output; y input
function z = fcn(x, y)
z = x(:) .* sign(y(:));

== matlab function sim_taes_2023_att/cal sig5 ==
  data: x input; z output; y input
function z = fcn(x, y)
z = x(:) .* sign(y(:));

== matlab function sim_taes_2023_att/trans to column10 ==
  data: x input; y output
function y = fcn(x)
y = x(:);

== matlab function sim_taes_2023_att/trans to column5 ==
  data: x input; y output
function y = fcn(x)
y = x(:);

== matlab function sim_taes_2023_att/trans to column6 ==
  data: x input; y output
function y = fcn(x)
y = x(:);

== matlab function sim_taes_2023_att/trans to column7 ==
  data: x input; y output
function y = fcn(x)
y = x(:);

== matlab function sim_taes_2023_att/trans to column8 ==
  data: x input; y output
function y = fcn(x)
y = x(:);

== matlab function sim_taes_2023_att/trans to column9 ==
  data: x input; y output
function y = fcn(x)
y = x(:);

== matlab function sim_taes_2023_att/choose ui agent 1 ==
  data: x input; y output
function y = fcn(x)
iiuav = 1;
y = x(:,iiuav);

== matlab function sim_taes_2023_att/cal d_theta_hat1 ==
  data: c1 input; d_ui_hat output; d_dui_hat output; d_d2ui_hat output; c2 input; c3 input; chi_t input; ui_sig_1 input; ui_sig_2 input; ui_sig_3 input; ui_sig_4 input; ui_sig_5 input; ui_sig_6 input; dui_hat input; d2ui_hat input
function [d_ui_hat, d_dui_hat, d_d2ui_hat] = fcn(c1, c2, c3, chi_t, ui_sig_1, ui_sig_2, ui_sig_3, ...
                                                                                        ui_sig_4, ui_sig_5, ui_sig_6, dui_hat, d2ui_hat)
d_d2ui_hat = -chi_t .* c1 * ui_sig_1(:) - (1 - chi_t) .* c1 * ui_sig_2(:);
d_dui_hat = -chi_t .* c2 * ui_sig_3(:) - (1 - chi_t) .* c2 * ui_sig_4(:) + d2ui_hat(:);
d_ui_hat = -chi_t .* c3 * ui_sig_5(:) - (1 - chi_t) .* c3 * ui_sig_6(:) + dui_hat(:);

== matlab function sim_taes_2023_att/cal sig10 ==
  data: x input; z output; y input
function z = fcn(x, y)
z = x(:) .* sign(y(:));

== matlab function sim_taes_2023_att/cal sig11 ==
  data: x input; z output; y input
function z = fcn(x, y)
z = x(:) .* sign(y(:));

== matlab function sim_taes_2023_att/cal sig6 ==
  data: x input; z output; y input
function z = fcn(x, y)
z = x(:) .* sign(y(:));

== matlab function sim_taes_2023_att/cal sig7 ==
  data: x input; z output; y input
function z = fcn(x, y)
z = x(:) .* sign(y(:));

== matlab function sim_taes_2023_att/cal sig8 ==
  data: x input; z output; y input
function z = fcn(x, y)
z = x(:) .* sign(y(:));

== matlab function sim_taes_2023_att/cal sig9 ==
  data: x input; z output; y input
function z = fcn(x, y)
z = x(:) .* sign(y(:));

== matlab function sim_taes_2023_att/choose ui agent 2 ==
  data: x input; y output
function y = fcn(x)
iiuav = 2;
y = x(:,iiuav);

== matlab function sim_taes_2023_att/trans to column11 ==
  data: x input; y output
function y = fcn(x)
y = x(:);

== matlab function sim_taes_2023_att/trans to column12 ==
  data: x input; y output
function y = fcn(x)
y = x(:);

== matlab function sim_taes_2023_att/trans to column13 ==
  data: x input; y output
function y = fcn(x)
y = x(:);

== matlab function sim_taes_2023_att/trans to column14 ==
  data: x input; y output
function y = fcn(x)
y = x(:);

== matlab function sim_taes_2023_att/trans to column15 ==
  data: x input; y output
function y = fcn(x)
y = x(:);

== matlab function sim_taes_2023_att/trans to column16 ==
  data: x input; y output
function y = fcn(x)
y = x(:);

== matlab function sim_taes_2023_att/cal d_theta_hat2 ==
  data: c1 input; d_ui_hat output; d_dui_hat output; d_d2ui_hat output; c2 input; c3 input; chi_t input; ui_sig_1 input; ui_sig_2 input; ui_sig_3 input; ui_sig_4 input; ui_sig_5 input; ui_sig_6 input; dui_hat input; d2ui_hat input
function [d_ui_hat, d_dui_hat, d_d2ui_hat] = fcn(c1, c2, c3, chi_t, ui_sig_1, ui_sig_2, ui_sig_3, ...
                                                                                        ui_sig_4, ui_sig_5, ui_sig_6, dui_hat, d2ui_hat)
d_d2ui_hat = -chi_t .* c1 * ui_sig_1(:) - (1 - chi_t) .* c1 * ui_sig_2(:);
d_dui_hat = -chi_t .* c2 * ui_sig_3(:) - (1 - chi_t) .* c2 * ui_sig_4(:) + d2ui_hat(:);
d_ui_hat = -chi_t .* c3 * ui_sig_5(:) - (1 - chi_t) .* c3 * ui_sig_6(:) + dui_hat(:);

== matlab function sim_taes_2023_att/cal sig12 ==
  data: x input; z output; y input
function z = fcn(x, y)
z = x(:) .* sign(y(:));

== matlab function sim_taes_2023_att/cal sig13 ==
  data: x input; z output; y input
function z = fcn(x, y)
z = x(:) .* sign(y(:));

== matlab function sim_taes_2023_att/cal sig14 ==
  data: x input; z output; y input
function z = fcn(x, y)
z = x(:) .* sign(y(:));

== matlab function sim_taes_2023_att/cal sig15 ==
  data: x input; z output; y input
function z = fcn(x, y)
z = x(:) .* sign(y(:));

== matlab function sim_taes_2023_att/cal sig16 ==
  data: x input; z output; y input
function z = fcn(x, y)
z = x(:) .* sign(y(:));

== matlab function sim_taes_2023_att/cal sig17 ==
  data: x input; z output; y input
function z = fcn(x, y)
z = x(:) .* sign(y(:));

== matlab function sim_taes_2023_att/choose ui agent 3 ==
  data: x input; y output
function y = fcn(x)
iiuav = 3;
y = x(:,iiuav);

== matlab function sim_taes_2023_att/trans to column17 ==
  data: x input; y output
function y = fcn(x)
y = x(:);

== matlab function sim_taes_2023_att/trans to column18 ==
  data: x input; y output
function y = fcn(x)
y = x(:);

== matlab function sim_taes_2023_att/trans to column19 ==
  data: x input; y output
function y = fcn(x)
y = x(:);

== matlab function sim_taes_2023_att/trans to column20 ==
  data: x input; y output
function y = fcn(x)
y = x(:);

== matlab function sim_taes_2023_att/trans to column21 ==
  data: x input; y output
function y = fcn(x)
y = x(:);

== matlab function sim_taes_2023_att/trans to column22 ==
  data: x input; y output
function y = fcn(x)
y = x(:);

== matlab function sim_taes_2023_att/cal d_theta_hat3 ==
  data: c1 input; d_ui_hat output; d_dui_hat output; d_d2ui_hat output; c2 input; c3 input; chi_t input; ui_sig_1 input; ui_sig_2 input; ui_sig_3 input; ui_sig_4 input; ui_sig_5 input; ui_sig_6 input; dui_hat input; d2ui_hat input
function [d_ui_hat, d_dui_hat, d_d2ui_hat] = fcn(c1, c2, c3, chi_t, ui_sig_1, ui_sig_2, ui_sig_3, ...
                                                                                        ui_sig_4, ui_sig_5, ui_sig_6, dui_hat, d2ui_hat)
d_d2ui_hat = -chi_t .* c1 * ui_sig_1(:) - (1 - chi_t) .* c1 * ui_sig_2(:);
d_dui_hat = -chi_t .* c2 * ui_sig_3(:) - (1 - chi_t) .* c2 * ui_sig_4(:) + d2ui_hat(:);
d_ui_hat = -chi_t .* c3 * ui_sig_5(:) - (1 - chi_t) .* c3 * ui_sig_6(:) + dui_hat(:);

== matlab function sim_taes_2023_att/cal sig18 ==
  data: x input; z output; y input
function z = fcn(x, y)
z = x(:) .* sign(y(:));

== matlab function sim_taes_2023_att/cal differentiator d_sigma_bar_w_hat agent 3/trans to column21 ==
  data: x input; y output
function y = fcn(x)
y = x(:);

== matlab function sim_taes_2023_att/cal sig19 ==
  data: x input; z output; y input
function z = fcn(x, y)
z = x(:) .* sign(y(:));

== matlab function sim_taes_2023_att/process velocity ==
  data: T0 input; T1 input; T2 input; PZ0 input; PZ1 input; R0 input; R1 input; Rx2 input; Ry2 input; Rz2 input; t input; V_init_out output
function V_init_out = fcn(T0, T1, T2, PZ0, PZ1, R0, R1, Rx2, Ry2, Rz2, t)
V_init_out = zeros(3, 1);
if t < T1 + 1e-05
    V_init_out(1, 1) = ( cos( ( 2 * pi * ( t - T0 ) ) / ( T0 - T1 ) ) * ( R0 - R1 ) ) / ( T0 - T1 ) ...
                                    - ( 2 * pi * sin( ( 2 * pi * ( t - T0 ) ) / ( T0 - T1 ) ) * ( R0 + ( ( R0 - R1 ) * ( t - T0 ) ) / ( T0 - T1 ) ) ) / ( T0 - T1 );
    V_init_out(2, 1) = ( sin( ( 2 * pi * ( t - T0 ) ) / ( T0 - T1 ) ) * ( R0 - R1 ) ) / ( T0 - T1 ) ...
                                    + ( 2 * pi * cos( ( 2 * pi * ( t - T0 ) ) / ( T0 - T1 ) ) * ( R0 + ( ( R0 - R1 ) * ( t - T0 ) ) / ( T0 - T1 ) ) ) / ( T0 - T1 );
    V_init_out(3, 1) = ( PZ0 - PZ1 ) / ( T0 - T1 );
else
    V_init_out(1, 1) = ( 2 * Rx2 * pi * sin( ( 2 * pi * ( t - T1 ) ) / ( T1 - T2 ) ) ) / ( T1 - T2 );
    V_init_out(2, 1) = ( 4 * Ry2 * pi * cos( ( 4 * pi * ( t - T1 ) ) / ( T1 - T2 ) ) ) / ( T1 - T2 );
    V_init_out(3, 1) = - ( 4 * Rz2 * pi * cos( ( 4 * pi * ( t - T1 ) ) / ( T1 - T2 ) ) ) / ( T1 - T2 );
end

== matlab function sim_taes_2023_att/cal sig20 ==
  data: x input; z output; y input
function z = fcn(x, y)
z = x(:) .* sign(y(:));

== matlab function sim_taes_2023_att/cal sig21 ==
  data: x input; z output; y input
function z = fcn(x, y)
z = x(:) .* sign(y(:));

== matlab function sim_taes_2023_att/cal sig22 ==
  data: x input; z output; y input
function z = fcn(x, y)
z = x(:) .* sign(y(:));

== matlab function sim_taes_2023_att/cal sig23 ==
  data: x input; z output; y input
function z = fcn(x, y)
z = x(:) .* sign(y(:));

== matlab function sim_taes_2023_att/choose ui agent 4 ==
  data: x input; y output
function y = fcn(x)
iiuav = 4;
y = x(:,iiuav);

== matlab function sim_taes_2023_att/trans to column23 ==
  data: x input; y output
function y = fcn(x)
y = x(:);

== matlab function sim_taes_2023_att/trans to column24 ==
  data: x input; y output
function y = fcn(x)
y = x(:);

== matlab function sim_taes_2023_att/trans to column25 ==
  data: x input; y output
function y = fcn(x)
y = x(:);

== matlab function sim_taes_2023_att/trans to column26 ==
  data: x input; y output
function y = fcn(x)
y = x(:);

== matlab function sim_taes_2023_att/trans to column27 ==
  data: x input; y output
function y = fcn(x)
y = x(:);

== matlab function sim_taes_2023_att/trans to column28 ==
  data: x input; y output
function y = fcn(x)
y = x(:);

== matlab function sim_taes_2023_att/cal d_theta_hat4 ==
  data: c1 input; d_ui_hat output; d_dui_hat output; d_d2ui_hat output; c2 input; c3 input; chi_t input; ui_sig_1 input; ui_sig_2 input; ui_sig_3 input; ui_sig_4 input; ui_sig_5 input; ui_sig_6 input; dui_hat input; d2ui_hat input
function [d_ui_hat, d_dui_hat, d_d2ui_hat] = fcn(c1, c2, c3, chi_t, ui_sig_1, ui_sig_2, ui_sig_3, ...
                                                                                        ui_sig_4, ui_sig_5, ui_sig_6, dui_hat, d2ui_hat)
d_d2ui_hat = -chi_t .* c1 * ui_sig_1(:) - (1 - chi_t) .* c1 * ui_sig_2(:);
d_dui_hat = -chi_t .* c2 * ui_sig_3(:) - (1 - chi_t) .* c2 * ui_sig_4(:) + d2ui_hat(:);
d_ui_hat = -chi_t .* c3 * ui_sig_5(:) - (1 - chi_t) .* c3 * ui_sig_6(:) + dui_hat(:);

== matlab function sim_taes_2023_att/cal sig24 ==
  data: x input; z output; y input
function z = fcn(x, y)
z = x(:) .* sign(y(:));

== matlab function sim_taes_2023_att/cal sig25 ==
  data: x input; z output; y input
function z = fcn(x, y)
z = x(:) .* sign(y(:));

== matlab function sim_taes_2023_att/cal sig26 ==
  data: x input; z output; y input
function z = fcn(x, y)
z = x(:) .* sign(y(:));

== matlab function sim_taes_2023_att/cal sig27 ==
  data: x input; z output; y input
function z = fcn(x, y)
z = x(:) .* sign(y(:));

== matlab function sim_taes_2023_att/cal sig28 ==
  data: x input; z output; y input
function z = fcn(x, y)
z = x(:) .* sign(y(:));
